simulink model "digitaltwin1c"  (R2020a)
settings: Solver=VariableStepAuto  StartTime=0.0  StopTime=stoptimetotal  RelTol=1e-3
values from neighbouring files (symbols this model uses):
  IC = load('params/IC_HoverAt10ftOcto.mat').IC    [prognostics.m]    (also in workspace_1.mat = )
  Motortwin1 = load('params/Motors/Motor1.mat').Motor    [prognostics.m]    (also in workspace_1.mat = )
  Motortwin2 = load('params/Motors/Motor2.mat').Motor    [prognostics.m]    (also in workspace_1.mat = )
  Motortwin3 = load('params/Motors/Motor3.mat').Motor    [prognostics.m]    (also in workspace_1.mat = )
  Motortwin4 = load('params/Motors/Motor4.mat').Motor    [prognostics.m]    (also in workspace_1.mat = )
  Motortwin5 = load('params/Motors/Motor5.mat').Motor    [prognostics.m]    (also in workspace_1.mat = )
  Motortwin6 = load('params/Motors/Motor6.mat').Motor    [prognostics.m]    (also in workspace_1.mat = )
  Motortwin7 = load('params/Motors/Motor7.mat').Motor    [prognostics.m]    (also in workspace_1.mat = )
  Motortwin8 = load('params/Motors/Motor8.mat').Motor    [prognostics.m]    (also in workspace_1.mat = )
  octomodel = load('params/octoModel.mat').octomodel    [prognostics.m]    (also in workspace_1.mat = )
  sampletimetraj = 1    [prognostics.m]    (also in workspace_1.mat)
undefined symbols (not defined in the file or in its folder): DiscIntNeverNeededParam, mu_wind
libraries: simulink x1, dspstat3 x1
(part 1 of 2)
settings Model: Creator=Researcher  LastModifiedBy=darrahts
settings DataIOCC: ReturnWorkspaceOutputs=off
settings DebuggingCC: ArithmeticOperatorsInVariantConditions=warning
settings SFSimCC: SimUseLocalCustomCode=off  CustomCodeUndefinedFunction=UseInterfaceOnly
settings RTWCC: RTWUseLocalCustomCode=off

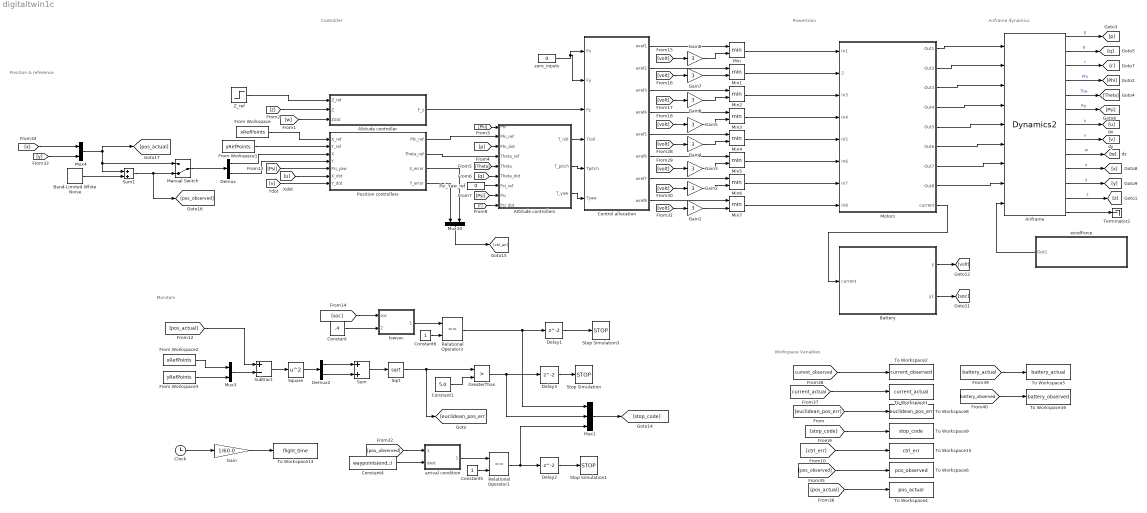
== system digitaltwin1c ==
  note: Workspace Variables
  note: Airframe dynamics
  note: Position & reference
  note: Controller
  note: Monitors
  note: Powertrain
  Airframe : M-S-Function  FunctionName=Dynamics2  Parameters=octomodel, IC
  Altitude controller : Subsystem
  Attitude controllers : Subsystem
  Band-Limited White Noise : simulink/Sources/Band-Limited White Noise  Cov=posNoise  Ts=sampletimetraj  seed=23
  Battery : Subsystem
  Clock : Clock
  Constant : Constant  Value=.4
  Constant1 : Constant  Value=5.0
  Constant4 : Constant  Value=waypoints(end,:)
  Constant5 : Constant
  Constant6 : Constant
  Control allocation : MATLAB Function  TreatAsAtomicUnit=on
  Delay1 : Delay
  Delay2 : Delay
  Delay3 : Delay
  Demux : Demux  Outputs=2
  Demux2 : Demux  Outputs=2
  From Workspace : FromWorkspace  VariableName=xRefPoints  SampleTime=sampletimetraj
  From Workspace1 : FromWorkspace  VariableName=yRefPoints  SampleTime=sampletimetraj
  From Workspace2 : FromWorkspace  VariableName=xRefPoints  SampleTime=sampletimetraj
  From Workspace3 : FromWorkspace  VariableName=yRefPoints  SampleTime=sampletimetraj
  Gain : Gain  Gain=1/60.0
  Gain{1..8} (8 alike) : Gain  Gain=3
  GreaterThan : RelationalOperator  Operator=>  OutDataTypeStr=boolean  RndMeth=Simplest
  Manual Switch : ManualSwitch  CurrentSetting=0
  Min{,1..7} (8 alike) : MinMax  Inputs=2
  Motors : Subsystem
  Mux1 : Mux  Inputs=3
  Mux10 : Mux  Inputs=2
  Mux3 : Mux  Inputs=2
  Mux4 : Mux  Inputs=2
  Position controllers : Subsystem
  Psi_Yaw_ref : Constant  Value=0
  Relational Operator1 : RelationalOperator  Operator===  OutDataTypeStr=boolean  RndMeth=Simplest
  Relational Operator3 : RelationalOperator  Operator===  OutDataTypeStr=boolean  RndMeth=Simplest
  Sqrt : Sqrt  SaturateOnIntegerOverflow=on
  Square : Math  Operator=square  SaturateOnIntegerOverflow=on
  Stop Simulation : Stop
  Stop Simulation1 : Stop
  Stop Simulation3 : Stop
  Subtract : Sum  Inputs=+-
  Sum : Sum
  Sum1 : Sum
  Terminator2 : Terminator
  To Workspace1 : ToWorkspace  VariableName=current_actual  SaveFormat=Timeseries  SampleTime=-1
  To Workspace13 : ToWorkspace  VariableName=flight_time  SaveFormat=Timeseries  SampleTime=-1
  To Workspace15 : ToWorkspace  VariableName=ctrl_err  SaveFormat=Timeseries  SampleTime=-1
  To Workspace16 : ToWorkspace  VariableName=battery_observed  SaveFormat=Timeseries  SampleTime=-1
  To Workspace2 : ToWorkspace  VariableName=current_observed  SaveFormat=Timeseries  SampleTime=-1
  To Workspace4 : ToWorkspace  VariableName=pos_actual  SaveFormat=Timeseries  SampleTime=-1
  To Workspace5 : ToWorkspace  VariableName=battery_actual  SaveFormat=Timeseries  SampleTime=-1
  To Workspace6 : ToWorkspace  VariableName=pos_observed  SaveFormat=Timeseries  SampleTime=-1
  To Workspace8 : ToWorkspace  VariableName=euclidean_pos_err  SaveFormat=Timeseries  SampleTime=-1
  To Workspace9 : ToWorkspace  VariableName=stop_code  SaveFormat=Timeseries  SampleTime=-1
  Z_ref : Step  Before=3  After=3  SampleTime=0
  arrival condition : MATLAB Function  TreatAsAtomicUnit=on
  lowsoc : MATLAB Function  TreatAsAtomicUnit=on
  windForce : Subsystem
  zero_inputs : Constant  Value=0
  wires:
  Airframe/1 -> [p]  "p"
  Airframe/2 -> [q]  "q"
  Airframe/3 -> [r]  "r"
  Airframe/4 -> [Phi]  "Phi"
  Airframe/5 -> [Theta]  "The"
  Airframe/6 -> [Psi]  "Psi"
  Airframe/11 -> [y]  "y"
  Airframe/12 -> [z]  "z"
  Airframe/7 -> [u]  "u"
  Airframe/10 -> [x]  "x"
  Airframe/9 -> [w]  "w"
  Airframe/8 -> [v]  "v"
  Motors/3(Out3) -> Airframe/3
  Motors/1(Out1) -> Airframe/1
  Motors/8(Out8) -> Airframe/8
  Motors/7(Out7) -> Airframe/7
  Motors/6(Out6) -> Airframe/6
  Motors/5(Out5) -> Airframe/5
  Motors/4(Out4) -> Airframe/4
  Motors/2(Out2) -> Airframe/2
  zero_inputs/1 -> Control allocation/1(Fx), Control allocation/2(Fy)
  Demux/2 -> Position controllers/4(Y)
  From Workspace1/1 -> Position controllers/2(Y_ref)
  From Workspace/1 -> Position controllers/1(X_ref)
  Demux/1 -> Position controllers/3(X)
  [Psi] -> Position controllers/5(Psi_yaw)
  [v] -> Position controllers/7(Y_dot)
  [u] -> Position controllers/6(X_dot)
  Position controllers/3(X_error) -> Mux10/2
  Position controllers/4(Y_error) -> Mux10/1
  Z_ref/1 -> Altitude controller/1(Z_ref)
  [z] -> Altitude controller/2(Z)
  Altitude controller/1(F_z) -> Control allocation/3(Fz)
  [Phi] -> Attitude controllers/1(Phi)
  [p] -> Attitude controllers/3(Phi_dot)
  Position controllers/2(Theta_ref) -> Attitude controllers/4(Theta_ref)
  [Theta] -> Attitude controllers/5(Theta)
  [q] -> Attitude controllers/6(Theta_dot)
  Psi_Yaw_ref/1 -> Attitude controllers/7(Psi_ref)
  [Psi] -> Attitude controllers/8(Psi)
  [r] -> Attitude controllers/9(Psi_dot)
  Attitude controllers/1(T_roll) -> Control allocation/4(Troll)
  Attitude controllers/2(T_pitch) -> Control allocation/5(Tpitch)
  Attitude controllers/3(T_yaw) -> Control allocation/6(Tyaw)
  Position controllers/1(Phi_ref) -> Attitude controllers/2(Phi_ref)
  [w] -> Altitude controller/3(Zdot)
  Airframe/13 -> Terminator2/1
  [volt] -> Gain1/1
  Min3/1 -> Motors/4(In4)
  Min4/1 -> Motors/5(In5)
  Min6/1 -> Motors/7(In7)
  Min7/1 -> Motors/8(In8)
  Control allocation/6(wref6) -> Min5/1
  Control allocation/7(wref7) -> Min6/1
  Gain4/1 -> Min4/2
  [volt] -> Gain8/1
  Min1/1 -> Motors/2(2)
  [volt] -> Gain3/1
  Control allocation/4(wref4) -> Min3/1
  [volt] -> Gain5/1
  [volt] -> Gain4/1
  Gain7/1 -> Min1/2
  Control allocation/2(wref2) -> Min1/1
  Gain5/1 -> Min3/2
  Min5/1 -> Motors/6(In6)
  Min2/1 -> Motors/3(In3)
  Min/1 -> Motors/1(In1)
  [volt] -> Gain6/1
  Control allocation/8(wref8) -> Min7/1
  Gain3/1 -> Min5/2
  [volt] -> Gain7/1
  Gain6/1 -> Min2/2
  Control allocation/1(wref1) -> Min/1
  Gain1/1 -> Min7/2
  Control allocation/3(wref3) -> Min2/1
  Gain2/1 -> Min6/2
  Gain8/1 -> Min/2
  [volt] -> Gain2/1
  Control allocation/5(wref5) -> Min4/1
  Mux4/1 -> [pos_actual], Manual Switch/1, Sum1/1
  [y] -> Mux4/2
  [x] -> Mux4/1
  Manual Switch/1 -> Demux/1
  Band-Limited White Noise/1 -> Sum1/2
  Sum1/1 -> [pos_observed], Manual Switch/2
  Clock/1 -> Gain/1
  Gain/1 -> To Workspace13/1
  Mux10/1 -> [ctrl_err]
  Motors/9(current) -> Battery/1(current)
  Battery/1(y) -> [volt]
  Battery/2(y1) -> [soc]
  windForce/1(Out1) -> Airframe/9
  Constant/1 -> lowsoc/2(threshold)
  From Workspace2/1 -> Mux3/1
  [soc] -> lowsoc/1(soc)
  Relational Operator1/1 -> Mux1/3, Delay2/1
  Sqrt/1 -> [euclidean_pos_err], GreaterThan/1
  Square/1 -> Demux2/1
  From Workspace3/1 -> Mux3/2
  Delay1/1 -> Stop Simulation3/1
  Mux1/1 -> [stop_code]
  Delay2/1 -> Stop Simulation1/1
  Constant1/1 -> GreaterThan/2
  GreaterThan/1 -> Mux1/2, Delay3/1
  Delay3/1 -> Stop Simulation/1
  [pos_observed] -> arrival condition/1(currentpos)
  Subtract/1 -> Square/1
  Demux2/2 -> Sum/2
  Constant6/1 -> Relational Operator3/2
  arrival condition/1(arrived) -> Relational Operator1/1
  Relational Operator3/1 -> Mux1/1, Delay1/1
  Sum/1 -> Sqrt/1
  Demux2/1 -> Sum/1
  Constant5/1 -> Relational Operator1/2
  Mux3/1 -> Subtract/2
  lowsoc/1(lowsoc) -> Relational Operator3/1
  [pos_actual] -> Subtract/1
  Constant4/1 -> arrival condition/2(dest)
  [euclidean_pos_err] -> To Workspace8/1
  [stop_code] -> To Workspace9/1
  [ctrl_err] -> To Workspace15/1
  [pos_observed] -> To Workspace6/1
  [pos_actual] -> To Workspace4/1
  [current_actual] -> To Workspace1/1
  [current_observed] -> To Workspace2/1
  [battery_actual] -> To Workspace5/1
  [battery_observed] -> To Workspace16/1

== system digitaltwin1c/Altitude controller ==
  Z_ref : Inport
  Z : Inport  Port=2
  Zdot : Inport  Port=3
  Add : Sum  Inputs=+++
  Add2 : Sum  Inputs=+-
  Constant2 : Constant  Value=octomodel.g*octomodel.mass
  Kdz : Gain  Gain=-3
  Kpz : Gain  Gain=-10
  mass : Gain  Gain=octomodel.mass
  mass1 : Gain  Gain=octomodel.mass
  F_z : Outport  VectorParamsAs1DForOutWhenUnconnected=off
  wires:
  Add2/1 -> Kpz/1
  Constant2/1 -> Add/1
  Z/1 -> Add2/1
  Add/1 -> F_z/1
  Z_ref/1 -> Add2/2
  Zdot/1 -> Kdz/1
  Kpz/1 -> mass/1
  Kdz/1 -> mass1/1
  mass1/1 -> Add/3
  mass/1 -> Add/2

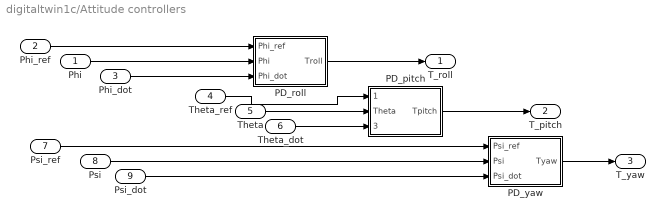
== system digitaltwin1c/Attitude controllers ==
  Phi : Inport
  Phi_ref : Inport  Port=2
  Phi_dot : Inport  Port=3
  Theta_ref : Inport  Port=4
  Theta : Inport  Port=5
  Theta_dot : Inport  Port=6
  Psi_ref : Inport  Port=7
  Psi : Inport  Port=8
  Psi_dot : Inport  Port=9
  PD_pitch : Subsystem
  PD_roll : Subsystem
  PD_yaw : Subsystem
  T_roll : Outport  VectorParamsAs1DForOutWhenUnconnected=off
  T_pitch : Outport  Port=2  VectorParamsAs1DForOutWhenUnconnected=off
  T_yaw : Outport  Port=3  VectorParamsAs1DForOutWhenUnconnected=off
  wires:
  PD_yaw/1(Tyaw) -> T_yaw/1
  PD_roll/1(Troll) -> T_roll/1
  Theta_ref/1 -> PD_pitch/1(Theta_ref)
  Theta_dot/1 -> PD_pitch/3(Theta_dot)
  PD_pitch/1(Tpitch) -> T_pitch/1
  Phi/1 -> PD_roll/2(Phi)
  Psi_dot/1 -> PD_yaw/3(Psi_dot)
  Psi_ref/1 -> PD_yaw/1(Psi_ref)
  Theta/1 -> PD_pitch/2(Theta)
  Phi_dot/1 -> PD_roll/3(Phi_dot)
  Psi/1 -> PD_yaw/2(Psi)
  Phi_ref/1 -> PD_roll/1(Phi_ref)

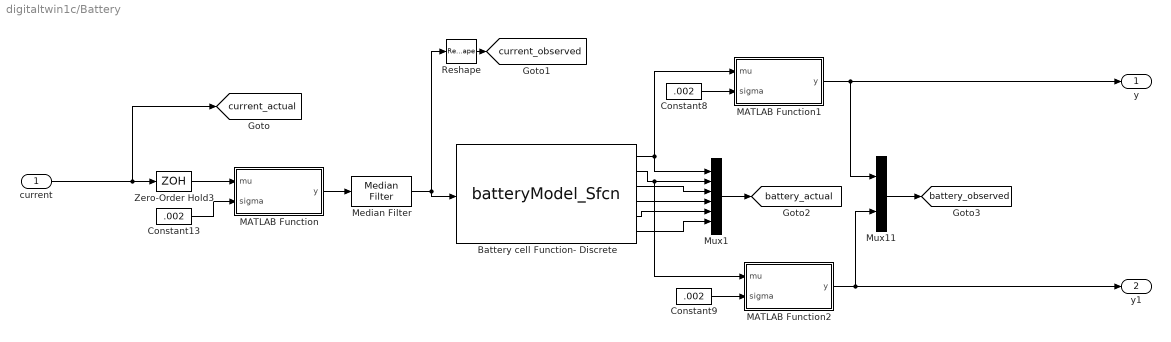
== system digitaltwin1c/Battery ==
  current : Inport
  Battery cell Function- Discrete : M-S-Function  FunctionName=batteryModel_Sfcn  Parameters=batterytwin, battery.dt
      mask Display:
      | port_label('input', 1, 'current');
      | port_label('output', 1, 'voltage');
      | port_label('output', 2, 'soc');
      | port_label('output', 3, 'R0');
      | port_label('output', 4, 'Ir');
      | port_label('output', 5, 'h');
      | port_label('output', 6, 'Q');
      | 
      | disp("Battery Cell");
  Constant13 : Constant  Value=.002
  Constant8 : Constant  Value=.002
  Constant9 : Constant  Value=.002
  MATLAB Function : MATLAB Function  TreatAsAtomicUnit=on
  MATLAB Function1 : MATLAB Function  TreatAsAtomicUnit=on
  MATLAB Function2 : MATLAB Function  TreatAsAtomicUnit=on
  Median Filter : dspstat3/Median Filter  WindowLength=5  SimulateUsing=Interpreted execution
      settings: SourceProductBaseCode=DS
  Mux1 : Mux  Inputs=6
  Mux11 : Mux  Inputs=2
  Reshape : Reshape
  Zero-Order Hold3 : ZeroOrderHold
  y : Outport
  y1 : Outport  Port=2
  tag scope: battery_actual=global, battery_observed=global, current_actual=global, current_observed=global
  wires:
  current/1 -> [current_actual], Zero-Order Hold3/1
  MATLAB Function/1(y) -> Median Filter/1
  Mux11/1 -> [battery_observed]
  MATLAB Function1/1(y) -> y/1, Mux11/1
  MATLAB Function2/1(y) -> y1/1, Mux11/2
  Battery cell Function- Discrete/1 -> MATLAB Function1/1(mu), Mux1/1
  Zero-Order Hold3/1 -> MATLAB Function/1(mu)
  Constant8/1 -> MATLAB Function1/2(sigma)
  Median Filter/1 -> Reshape/1, Battery cell Function- Discrete/1
  Battery cell Function- Discrete/2 -> MATLAB Function2/1(mu), Mux1/2
  Mux1/1 -> [battery_actual]
  Constant13/1 -> MATLAB Function/2(sigma)
  Constant9/1 -> MATLAB Function2/2(sigma)
  Battery cell Function- Discrete/3 -> Mux1/3
  Battery cell Function- Discrete/4 -> Mux1/4
  Battery cell Function- Discrete/5 -> Mux1/5
  Battery cell Function- Discrete/6 -> Mux1/6
  Reshape/1 -> [current_observed]

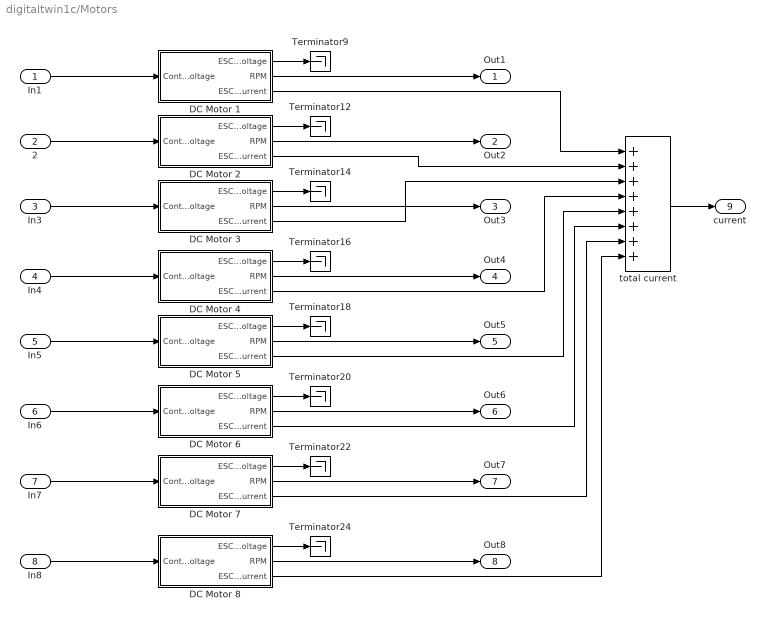
== system digitaltwin1c/Motors ==
  In1 : Inport
  2 : Inport  Port=2
  In3 : Inport  Port=3
  In4 : Inport  Port=4
  In5 : Inport  Port=5
  In6 : Inport  Port=6
  In7 : Inport  Port=7
  In8 : Inport  Port=8
  "DC Motor 1 " : Subsystem
  DC Motor 2 : Subsystem
  DC Motor 3 : Subsystem
  DC Motor 4 : Subsystem
  DC Motor 5 : Subsystem
  DC Motor 6 : Subsystem
  DC Motor 7 : Subsystem
  DC Motor 8 : Subsystem
  Terminator{9,12,14,16,18,20,22,24} (8 alike) : Terminator
  total current : Sum  Inputs=++++++++
  Out1 : Outport  VectorParamsAs1DForOutWhenUnconnected=off
  Out2 : Outport  Port=2  VectorParamsAs1DForOutWhenUnconnected=off
  Out3 : Outport  Port=3  VectorParamsAs1DForOutWhenUnconnected=off
  Out4 : Outport  Port=4  VectorParamsAs1DForOutWhenUnconnected=off
  Out5 : Outport  Port=5  VectorParamsAs1DForOutWhenUnconnected=off
  Out6 : Outport  Port=6  VectorParamsAs1DForOutWhenUnconnected=off
  Out7 : Outport  Port=7  VectorParamsAs1DForOutWhenUnconnected=off
  Out8 : Outport  Port=8  VectorParamsAs1DForOutWhenUnconnected=off
  current : Outport  Port=9  VectorParamsAs1DForOutWhenUnconnected=off
  wires:
  DC Motor 5/1(ESC Voltage) -> Terminator18/1
  DC Motor 6/3(ESC Current) -> total current/6
  DC Motor 7/3(ESC Current) -> total current/7
  DC Motor 7/1(ESC Voltage) -> Terminator22/1
  DC Motor 6/1(ESC Voltage) -> Terminator20/1
  DC Motor 5/3(ESC Current) -> total current/5
  DC Motor 8/3(ESC Current) -> total current/8
  "DC Motor 1 "/3(ESC Current) -> total current/1
  "DC Motor 1 "/1(ESC Voltage) -> Terminator9/1
  DC Motor 2/3(ESC Current) -> total current/2
  DC Motor 2/1(ESC Voltage) -> Terminator12/1
  DC Motor 3/1(ESC Voltage) -> Terminator14/1
  DC Motor 4/3(ESC Current) -> total current/4
  DC Motor 3/3(ESC Current) -> total current/3
  DC Motor 5/2(RPM) -> Out5/1
  DC Motor 4/1(ESC Voltage) -> Terminator16/1
  DC Motor 8/1(ESC Voltage) -> Terminator24/1
  DC Motor 7/2(RPM) -> Out7/1
  DC Motor 2/2(RPM) -> Out2/1
  DC Motor 3/2(RPM) -> Out3/1
  DC Motor 4/2(RPM) -> Out4/1
  DC Motor 6/2(RPM) -> Out6/1
  DC Motor 8/2(RPM) -> Out8/1
  "DC Motor 1 "/2(RPM) -> Out1/1
  In1/1 -> "DC Motor 1 "/1(Control  Voltage)
  In7/1 -> DC Motor 7/1(Control  Voltage)
  In8/1 -> DC Motor 8/1(Control  Voltage)
  In6/1 -> DC Motor 6/1(Control  Voltage)
  In5/1 -> DC Motor 5/1(Control  Voltage)
  In4/1 -> DC Motor 4/1(Control  Voltage)
  In3/1 -> DC Motor 3/1(Control  Voltage)
  2/1 -> DC Motor 2/1(Control  Voltage)
  total current/1 -> current/1

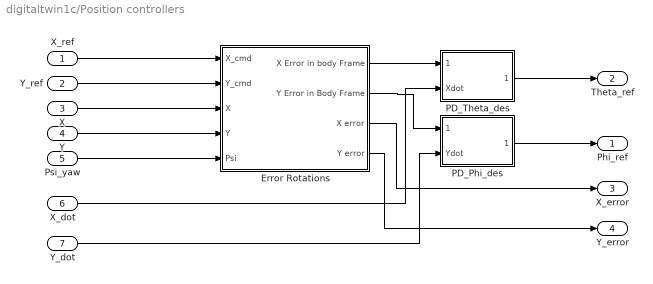
== system digitaltwin1c/Position controllers ==
  X_ref : Inport
  Y_ref : Inport  Port=2
  X : Inport  Port=3
  Y : Inport  Port=4
  Psi_yaw : Inport  Port=5
  X_dot : Inport  Port=6
  Y_dot : Inport  Port=7
  Error Rotations : Subsystem
  PD_Phi_des : Subsystem
  PD_Theta_des : Subsystem
  Phi_ref : Outport  VectorParamsAs1DForOutWhenUnconnected=off
  Theta_ref : Outport  Port=2  VectorParamsAs1DForOutWhenUnconnected=off
  X_error : Outport  Port=3  VectorParamsAs1DForOutWhenUnconnected=off
  Y_error : Outport  Port=4  VectorParamsAs1DForOutWhenUnconnected=off
  wires:
  Y/1 -> Error Rotations/4(Y)
  Y_ref/1 -> Error Rotations/2(Y_cmd)
  Error Rotations/4("Y error ") -> Y_error/1
  Error Rotations/3(X error) -> X_error/1
  Error Rotations/1(X Error in body Frame) -> PD_Theta_des/1(Xdot_ref)
  X/1 -> Error Rotations/3(X)
  Y_dot/1 -> PD_Phi_des/2(Ydot)
  PD_Phi_des/1(Phi_des) -> Phi_ref/1
  Error Rotations/2(Y Error in Body Frame) -> PD_Phi_des/1(Ydot_ref)
  Psi_yaw/1 -> Error Rotations/5(Psi)
  PD_Theta_des/1(Theta_des) -> Theta_ref/1
  X_dot/1 -> PD_Theta_des/2(Xdot)
  X_ref/1 -> Error Rotations/1(X_cmd)

== system digitaltwin1c/windForce ==
  Constant10 : Constant  Value=[0;0;0]
  Gain : Gain  Gain=.5
  Manual Switch1 : ManualSwitch  CurrentSetting=0
  Mux9 : Mux  Inputs=3
  Random Number : RandomNumber  Mean=mu_wind  Variance=.5  Seed=37
  Random Number1 : RandomNumber  Mean=mu_wind  Variance=.5  Seed=41
  Random Number2 : RandomNumber  Mean=mu_wind  Variance=.5
  Out1 : Outport
  wires:
  Random Number1/1 -> Mux9/2
  Mux9/1 -> Gain/1
  Manual Switch1/1 -> Out1/1
  Random Number2/1 -> Mux9/3
  Random Number/1 -> Mux9/1
  Constant10/1 -> Manual Switch1/1
  Gain/1 -> Manual Switch1/2

== system digitaltwin1c/Attitude controllers/PD_pitch ==
  Theta_ref : Inport
  Theta : Inport  Port=2
  Theta_dot : Inport  Port=3
  Add : Sum  Inputs=-+
  Gain : Gain  Gain=3
  Gain1 : Gain
  Gain2 : Gain  Gain=-1
  Sum : Sum  Inputs=|++
  Tpitch : Outport  VectorParamsAs1DForOutWhenUnconnected=off
  wires:
  Gain2/1 -> Tpitch/1
  Gain/1 -> Sum/1
  Theta/1 -> Add/2
  Add/1 -> Gain/1
  Gain1/1 -> Sum/2
  Sum/1 -> Gain2/1
  Theta_dot/1 -> Gain1/1
  Theta_ref/1 -> Add/1

== system digitaltwin1c/Attitude controllers/PD_roll ==
  Phi_ref : Inport
  Phi : Inport  Port=2
  Phi_dot : Inport  Port=3
  Add : Sum  Inputs=-+
  Gain : Gain  Gain=3
  Gain1 : Gain
  Gain2 : Gain  Gain=-1
  Sum : Sum  Inputs=|++
  Troll : Outport  VectorParamsAs1DForOutWhenUnconnected=off
  wires:
  Phi_ref/1 -> Add/1
  Phi_dot/1 -> Gain1/1
  Sum/1 -> Gain2/1
  Gain1/1 -> Sum/2
  Add/1 -> Gain/1
  Phi/1 -> Add/2
  Gain/1 -> Sum/1
  Gain2/1 -> Troll/1

== system digitaltwin1c/Attitude controllers/PD_yaw ==
  Psi_ref : Inport
  Psi : Inport  Port=2
  Psi_dot : Inport  Port=3
  Add : Sum  Inputs=-+
  Gain : Gain  Gain=3
  Gain1 : Gain
  Gain2 : Gain  Gain=-1
  Sum : Sum  Inputs=|++
  Tyaw : Outport  VectorParamsAs1DForOutWhenUnconnected=off
  wires:
  Psi_ref/1 -> Add/1
  Psi_dot/1 -> Gain1/1
  Sum/1 -> Gain2/1
  Gain1/1 -> Sum/2
  Add/1 -> Gain/1
  Psi/1 -> Add/2
  Gain/1 -> Sum/1
  Gain2/1 -> Tyaw/1

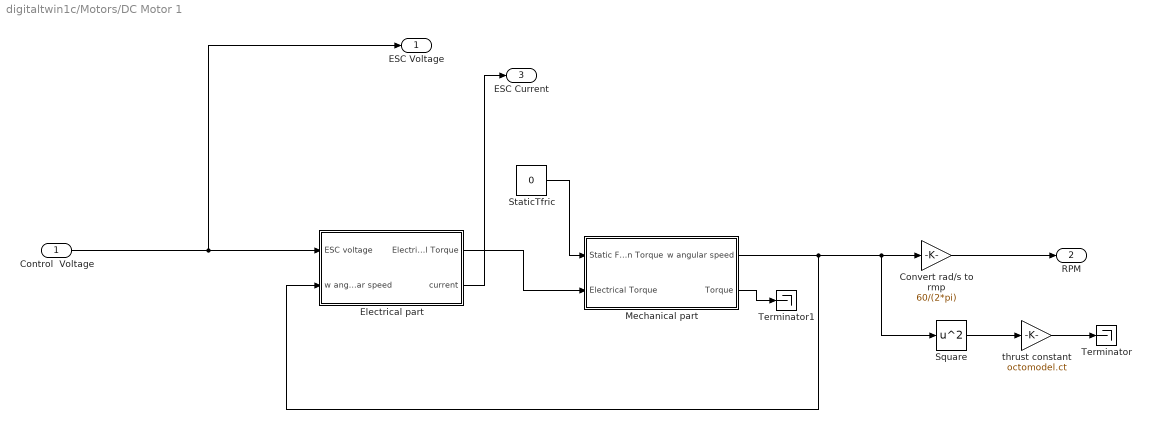
== system digitaltwin1c/Motors/DC Motor 1  ==
  Control  Voltage : Inport
  Convert rad/s to rmp : Gain  Gain=60/(2*pi)
  Electrical part : Subsystem
  Mechanical part : Subsystem
  Square : Math  Operator=square  SaturateOnIntegerOverflow=on
  StaticTfric : Constant  Value=0
  Terminator : Terminator
  Terminator1 : Terminator
  thrust constant : Gain  Gain=octomodel.ct
  ESC Voltage : Outport  VectorParamsAs1DForOutWhenUnconnected=off
  RPM : Outport  Port=2  VectorParamsAs1DForOutWhenUnconnected=off
  ESC Current : Outport  Port=3  VectorParamsAs1DForOutWhenUnconnected=off
  wires:
  Electrical part/1(Electrical Torque) -> Mechanical part/2(Electrical Torque)
  StaticTfric/1 -> Mechanical part/1(Static Friction Torque)
  Control  Voltage/1 -> ESC Voltage/1, Electrical part/1(ESC voltage)
  Electrical part/2(current) -> ESC Current/1
  Convert rad/s to rmp/1 -> RPM/1
  Mechanical part/1(w angular speed) -> Electrical part/2(w angular speed), Square/1, Convert rad/s to rmp/1
  Square/1 -> thrust constant/1
  thrust constant/1 -> Terminator/1
  Mechanical part/2(Torque) -> Terminator1/1

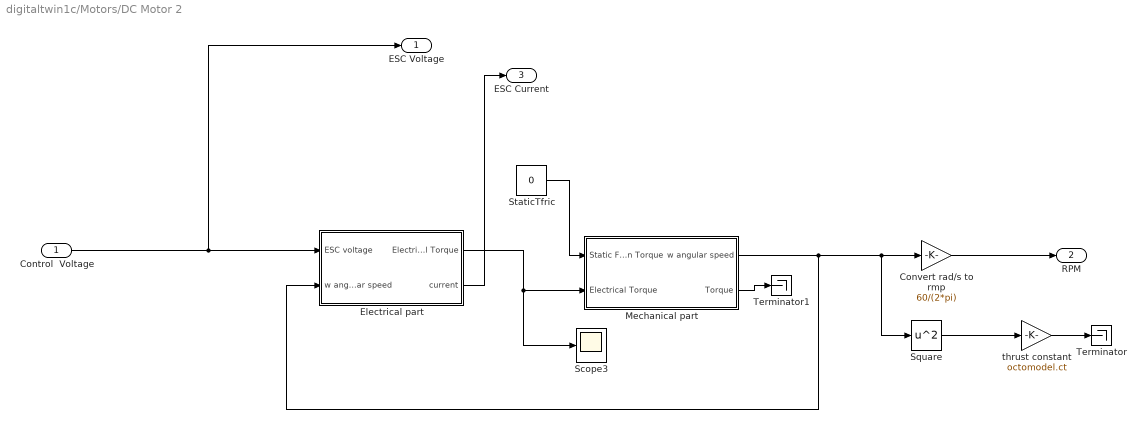
== system digitaltwin1c/Motors/DC Motor 2 ==
  Control  Voltage : Inport
  Convert rad/s to rmp : Gain  Gain=60/(2*pi)
  Electrical part : Subsystem
  Mechanical part : Subsystem
  Scope3 : Scope
  Square : Math  Operator=square  SaturateOnIntegerOverflow=on
  StaticTfric : Constant  Value=0
  Terminator : Terminator
  Terminator1 : Terminator
  thrust constant : Gain  Gain=octomodel.ct
  ESC Voltage : Outport  VectorParamsAs1DForOutWhenUnconnected=off
  RPM : Outport  Port=2  VectorParamsAs1DForOutWhenUnconnected=off
  ESC Current : Outport  Port=3  VectorParamsAs1DForOutWhenUnconnected=off
  wires:
  Square/1 -> thrust constant/1
  Mechanical part/1(w angular speed) -> Convert rad/s to rmp/1, Square/1, Electrical part/2(w angular speed)
  Convert rad/s to rmp/1 -> RPM/1
  Electrical part/2(current) -> ESC Current/1
  Control  Voltage/1 -> Electrical part/1(ESC voltage), ESC Voltage/1
  StaticTfric/1 -> Mechanical part/1(Static Friction Torque)
  Electrical part/1(Electrical Torque) -> Mechanical part/2(Electrical Torque), Scope3/1
  thrust constant/1 -> Terminator/1
  Mechanical part/2(Torque) -> Terminator1/1

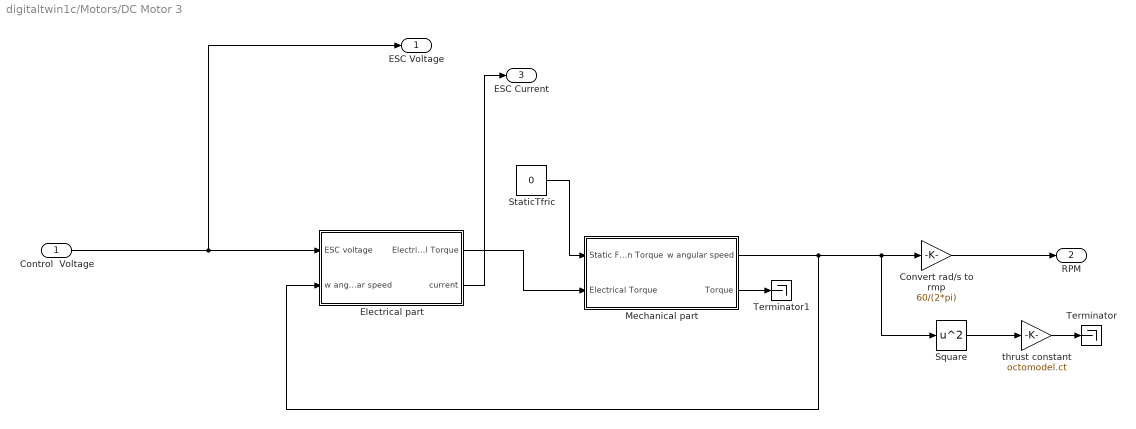
== system digitaltwin1c/Motors/DC Motor 3 ==
  Control  Voltage : Inport
  Convert rad/s to rmp : Gain  Gain=60/(2*pi)
  Electrical part : Subsystem
  Mechanical part : Subsystem
  Square : Math  Operator=square  SaturateOnIntegerOverflow=on
  StaticTfric : Constant  Value=0
  Terminator : Terminator
  Terminator1 : Terminator
  thrust constant : Gain  Gain=octomodel.ct
  ESC Voltage : Outport  VectorParamsAs1DForOutWhenUnconnected=off
  RPM : Outport  Port=2  VectorParamsAs1DForOutWhenUnconnected=off
  ESC Current : Outport  Port=3  VectorParamsAs1DForOutWhenUnconnected=off
  wires:
  Electrical part/1(Electrical Torque) -> Mechanical part/2(Electrical Torque)
  StaticTfric/1 -> Mechanical part/1(Static Friction Torque)
  Control  Voltage/1 -> ESC Voltage/1, Electrical part/1(ESC voltage)
  Electrical part/2(current) -> ESC Current/1
  Convert rad/s to rmp/1 -> RPM/1
  Mechanical part/1(w angular speed) -> Electrical part/2(w angular speed), Square/1, Convert rad/s to rmp/1
  Square/1 -> thrust constant/1
  thrust constant/1 -> Terminator/1
  Mechanical part/2(Torque) -> Terminator1/1

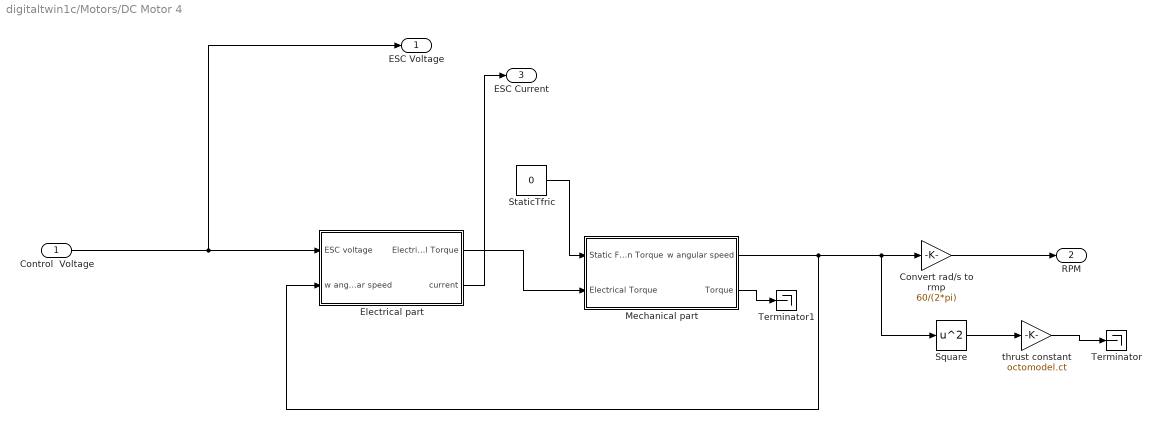
== system digitaltwin1c/Motors/DC Motor 4 ==
  Control  Voltage : Inport
  Convert rad/s to rmp : Gain  Gain=60/(2*pi)
  Electrical part : Subsystem
  Mechanical part : Subsystem
  Square : Math  Operator=square  SaturateOnIntegerOverflow=on
  StaticTfric : Constant  Value=0
  Terminator : Terminator
  Terminator1 : Terminator
  thrust constant : Gain  Gain=octomodel.ct
  ESC Voltage : Outport  VectorParamsAs1DForOutWhenUnconnected=off
  RPM : Outport  Port=2  VectorParamsAs1DForOutWhenUnconnected=off
  ESC Current : Outport  Port=3  VectorParamsAs1DForOutWhenUnconnected=off
  wires:
  Square/1 -> thrust constant/1
  Mechanical part/1(w angular speed) -> Convert rad/s to rmp/1, Square/1, Electrical part/2(w angular speed)
  Convert rad/s to rmp/1 -> RPM/1
  Electrical part/2(current) -> ESC Current/1
  Control  Voltage/1 -> Electrical part/1(ESC voltage), ESC Voltage/1
  StaticTfric/1 -> Mechanical part/1(Static Friction Torque)
  Electrical part/1(Electrical Torque) -> Mechanical part/2(Electrical Torque)
  thrust constant/1 -> Terminator/1
  Mechanical part/2(Torque) -> Terminator1/1

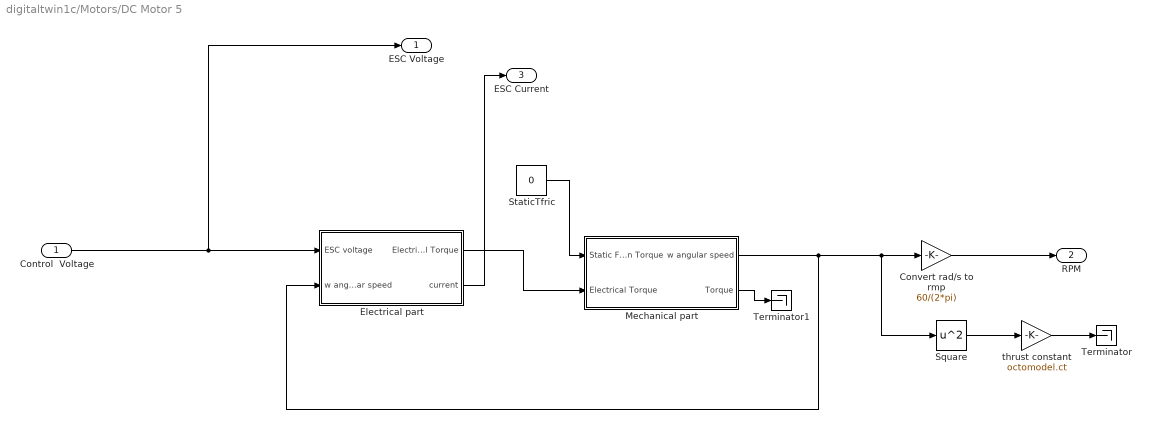
== system digitaltwin1c/Motors/DC Motor 5 ==
  Control  Voltage : Inport
  Convert rad/s to rmp : Gain  Gain=60/(2*pi)
  Electrical part : Subsystem
  Mechanical part : Subsystem
  Square : Math  Operator=square  SaturateOnIntegerOverflow=on
  StaticTfric : Constant  Value=0
  Terminator : Terminator
  Terminator1 : Terminator
  thrust constant : Gain  Gain=octomodel.ct
  ESC Voltage : Outport  VectorParamsAs1DForOutWhenUnconnected=off
  RPM : Outport  Port=2  VectorParamsAs1DForOutWhenUnconnected=off
  ESC Current : Outport  Port=3  VectorParamsAs1DForOutWhenUnconnected=off
  wires:
  Electrical part/1(Electrical Torque) -> Mechanical part/2(Electrical Torque)
  StaticTfric/1 -> Mechanical part/1(Static Friction Torque)
  Control  Voltage/1 -> ESC Voltage/1, Electrical part/1(ESC voltage)
  Electrical part/2(current) -> ESC Current/1
  Convert rad/s to rmp/1 -> RPM/1
  Mechanical part/1(w angular speed) -> Electrical part/2(w angular speed), Square/1, Convert rad/s to rmp/1
  Square/1 -> thrust constant/1
  thrust constant/1 -> Terminator/1
  Mechanical part/2(Torque) -> Terminator1/1

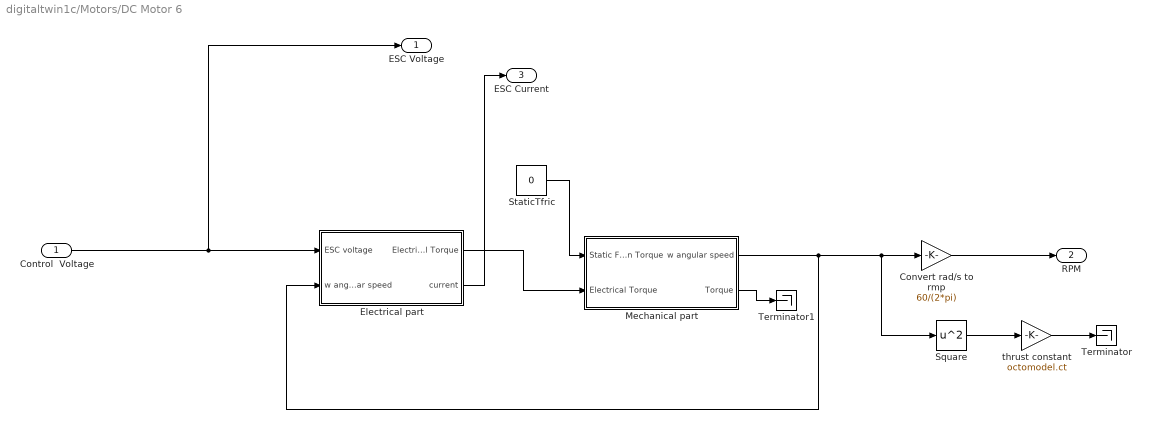
== system digitaltwin1c/Motors/DC Motor 6 ==
  Control  Voltage : Inport
  Convert rad/s to rmp : Gain  Gain=60/(2*pi)
  Electrical part : Subsystem
  Mechanical part : Subsystem
  Square : Math  Operator=square  SaturateOnIntegerOverflow=on
  StaticTfric : Constant  Value=0
  Terminator : Terminator
  Terminator1 : Terminator
  thrust constant : Gain  Gain=octomodel.ct
  ESC Voltage : Outport  VectorParamsAs1DForOutWhenUnconnected=off
  RPM : Outport  Port=2  VectorParamsAs1DForOutWhenUnconnected=off
  ESC Current : Outport  Port=3  VectorParamsAs1DForOutWhenUnconnected=off
  wires:
  Square/1 -> thrust constant/1
  Mechanical part/1(w angular speed) -> Convert rad/s to rmp/1, Square/1, Electrical part/2(w angular speed)
  Convert rad/s to rmp/1 -> RPM/1
  Electrical part/2(current) -> ESC Current/1
  Control  Voltage/1 -> Electrical part/1(ESC voltage), ESC Voltage/1
  StaticTfric/1 -> Mechanical part/1(Static Friction Torque)
  Electrical part/1(Electrical Torque) -> Mechanical part/2(Electrical Torque)
  thrust constant/1 -> Terminator/1
  Mechanical part/2(Torque) -> Terminator1/1

== system digitaltwin1c/Motors/DC Motor 7 ==
  Control  Voltage : Inport
  Convert rad/s to rmp : Gain  Gain=60/(2*pi)
  Electrical part : Subsystem
  Mechanical part : Subsystem
  Square : Math  Operator=square  SaturateOnIntegerOverflow=on
  StaticTfric : Constant  Value=0
  Terminator : Terminator
  Terminator1 : Terminator
  thrust constant : Gain  Gain=octomodel.ct
  ESC Voltage : Outport  VectorParamsAs1DForOutWhenUnconnected=off
  RPM : Outport  Port=2  VectorParamsAs1DForOutWhenUnconnected=off
  ESC Current : Outport  Port=3  VectorParamsAs1DForOutWhenUnconnected=off
  wires:
  Electrical part/1(Electrical Torque) -> Mechanical part/2(Electrical Torque)
  StaticTfric/1 -> Mechanical part/1(Static Friction Torque)
  Control  Voltage/1 -> ESC Voltage/1, Electrical part/1(ESC voltage)
  Electrical part/2(current) -> ESC Current/1
  Convert rad/s to rmp/1 -> RPM/1
  Mechanical part/1(w angular speed) -> Electrical part/2(w angular speed), Square/1, Convert rad/s to rmp/1
  Square/1 -> thrust constant/1
  thrust constant/1 -> Terminator/1
  Mechanical part/2(Torque) -> Terminator1/1

== system digitaltwin1c/Motors/DC Motor 8 ==
  Control  Voltage : Inport
  Convert rad/s to rmp : Gain  Gain=60/(2*pi)
  Electrical part : Subsystem
  Mechanical part : Subsystem
  Square : Math  Operator=square  SaturateOnIntegerOverflow=on
  StaticTfric : Constant  Value=0
  Terminator : Terminator
  Terminator1 : Terminator
  thrust constant : Gain  Gain=octomodel.ct
  ESC Voltage : Outport  VectorParamsAs1DForOutWhenUnconnected=off
  RPM : Outport  Port=2  VectorParamsAs1DForOutWhenUnconnected=off
  ESC Current : Outport  Port=3  VectorParamsAs1DForOutWhenUnconnected=off
  wires:
  Square/1 -> thrust constant/1
  Mechanical part/1(w angular speed) -> Convert rad/s to rmp/1, Square/1, Electrical part/2(w angular speed)
  Convert rad/s to rmp/1 -> RPM/1
  Electrical part/2(current) -> ESC Current/1
  Control  Voltage/1 -> Electrical part/1(ESC voltage), ESC Voltage/1
  StaticTfric/1 -> Mechanical part/1(Static Friction Torque)
  Electrical part/1(Electrical Torque) -> Mechanical part/2(Electrical Torque)
  thrust constant/1 -> Terminator/1
  Mechanical part/2(Torque) -> Terminator1/1

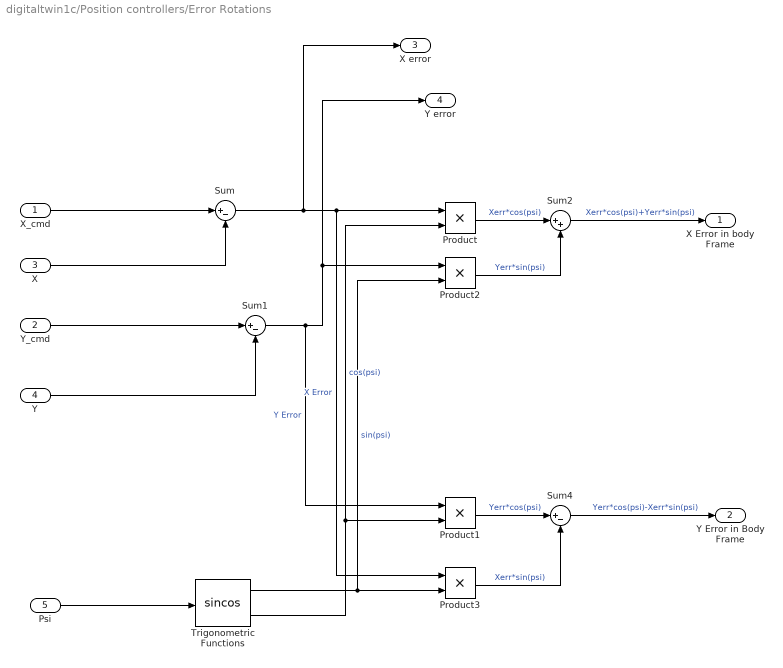
== system digitaltwin1c/Position controllers/Error Rotations ==
  X_cmd : Inport
  Y_cmd : Inport  Port=2
  X : Inport  Port=3
  Y : Inport  Port=4
  Psi : Inport  Port=5
  Product{,1..3} (4 alike) : Product
  Sum : Sum  Inputs=|+-
  Sum1 : Sum  Inputs=|+-
  Sum2 : Sum  Inputs=|++
  Sum4 : Sum  Inputs=|+-
  Trigonometric Functions : Trigonometry  Operator=sincos
  X Error in body Frame : Outport  VectorParamsAs1DForOutWhenUnconnected=off
  Y Error in Body Frame : Outport  Port=2  VectorParamsAs1DForOutWhenUnconnected=off
  X error : Outport  Port=3  VectorParamsAs1DForOutWhenUnconnected=off
  "Y error " : Outport  Port=4  VectorParamsAs1DForOutWhenUnconnected=off
  wires:
  Sum4/1 -> Y Error in Body Frame/1  "Yerr*cos(psi)-Xerr*sin(psi)"
  Product3/1 -> Sum4/2  "Xerr*sin(psi)"
  Sum1/1 -> "Y error "/1, Product2/1, Product1/1  "Y Error"
  Trigonometric Functions/1 -> Product2/2, Product3/2  "sin(psi)"
  Sum2/1 -> X Error in body Frame/1  "Xerr*cos(psi)+Yerr*sin(psi)"
  Y_cmd/1 -> Sum1/1
  X_cmd/1 -> Sum/1
  X/1 -> Sum/2
  Y/1 -> Sum1/2
  Sum/1 -> X error/1, Product3/1, Product/1  "X Error"
  Trigonometric Functions/2 -> Product/2, Product1/2  "cos(psi)"
  Product/1 -> Sum2/1  "Xerr*cos(psi)"
  Product2/1 -> Sum2/2  "Yerr*sin(psi)"
  Product1/1 -> Sum4/1  "Yerr*cos(psi)"
  Psi/1 -> Trigonometric Functions/1

== system digitaltwin1c/Position controllers/PD_Phi_des ==
  Ydot_ref : Inport
  Ydot : Inport  Port=2
  Add : Sum  Inputs=+-
  Gain : Gain  Gain=0.1
  Gain1 : Gain  Gain=0
  Gain2 : Gain  Gain=-1
  Saturation in radians : Saturate  UpperLimit=12*pi/180  LowerLimit=-12*pi/180
  Sum : Sum  Inputs=|+-
  Phi_des : Outport  VectorParamsAs1DForOutWhenUnconnected=off
  wires:
  Saturation in radians/1 -> Phi_des/1
  Ydot_ref/1 -> Add/1
  Ydot/1 -> Add/2, Gain1/1
  Gain1/1 -> Sum/2
  Add/1 -> Gain/1
  Gain/1 -> Sum/1
  Sum/1 -> Gain2/1
  Gain2/1 -> Saturation in radians/1

== system digitaltwin1c/Position controllers/PD_Theta_des ==
  Xdot_ref : Inport
  Xdot : Inport  Port=2
  Add : Sum  Inputs=+-
  Gain : Gain  Gain=0.1
  Gain1 : Gain  Gain=0
  Saturation in radians : Saturate  UpperLimit=12*pi/180  LowerLimit=-12*pi/180
  Sum : Sum  Inputs=|+-
  Theta_des : Outport  VectorParamsAs1DForOutWhenUnconnected=off
  wires:
  Sum/1 -> Saturation in radians/1
  Gain/1 -> Sum/1
  Add/1 -> Gain/1
  Gain1/1 -> Sum/2
  Xdot/1 -> Gain1/1, Add/2
  Xdot_ref/1 -> Add/1
  Saturation in radians/1 -> Theta_des/1

== system digitaltwin1c/Motors/DC Motor 1 /Electrical part ==
  ESC voltage : Inport
  w angular speed : Inport  Port=2
  1/R : Gain  Gain=1/Motortwin1.Req
  Ke (Torque constant)1 : Gain  Gain=Motortwin1.Ke_eq
  Kt (Torque constant) Kt=Ke for an ideal square wave motor : Gain  Gain=Motortwin1.Ke_eq
  Saturation : Saturate  UpperLimit=11  LowerLimit=0
  Sum : Sum  Inputs=|+-
  Electrical Torque : Outport  VectorParamsAs1DForOutWhenUnconnected=off
  current : Outport  Port=2  VectorParamsAs1DForOutWhenUnconnected=off
  wires:
  1/R/1 -> Saturation/1  "current i"
  Sum/1 -> 1/R/1
  Kt (Torque constant) Kt=Ke for an ideal square wave motor/1 -> Electrical Torque/1
  Ke (Torque constant)1/1 -> Sum/2
  ESC voltage/1 -> Sum/1
  w angular speed/1 -> Ke (Torque constant)1/1
  Saturation/1 -> Kt (Torque constant) Kt=Ke for an ideal square wave motor/1, current/1

== system digitaltwin1c/Motors/DC Motor 1 /Mechanical part ==
  Static Friction Torque : Inport
  Electrical Torque : Inport  Port=2
  1/J Inertia constant : Gain  Gain=1/Motortwin1.J
  "Df viscous damping coefficient Dynamic Friction coefficient " : Gain  Gain=Motortwin1.Df
  Discrete-Time Integrator : DiscreteIntegrator  gainval=1  InitialCondition=IC.w1  SampleTime=octomodel.sampletime  ICPrevOutput=DiscIntNeverNeededParam  ICPrevScaledInput=DiscIntNeverNeededParam
  Gain : Gain  Gain=Motortwin1.cq
  Square : Math  Operator=square  SaturateOnIntegerOverflow=on
  Sum1 : Sum  Inputs=--+-
  w angular speed : Outport  VectorParamsAs1DForOutWhenUnconnected=off
  Torque : Outport  Port=2  VectorParamsAs1DForOutWhenUnconnected=off
  wires:
  1/J Inertia constant/1 -> Discrete-Time Integrator/1
  Static Friction Torque/1 -> Sum1/2
  "Df viscous damping coefficient Dynamic Friction coefficient "/1 -> Sum1/4
  Discrete-Time Integrator/1 -> w angular speed/1, Square/1, "Df viscous damping coefficient Dynamic Friction coefficient "/1  "w angular speed"
  Sum1/1 -> 1/J Inertia constant/1
  Electrical Torque/1 -> Sum1/3
  Gain/1 -> Torque/1, Sum1/1
  Square/1 -> Gain/1

== system digitaltwin1c/Motors/DC Motor 2/Electrical part ==
  ESC voltage : Inport
  w angular speed : Inport  Port=2
  1/R : Gain  Gain=1/Motortwin2.Req
  Ke (Torque constant)1 : Gain  Gain=Motortwin2.Ke_eq
  Kt (Torque constant) Kt=Ke for an ideal square wave motor : Gain  Gain=Motortwin2.Ke_eq
  Saturation : Saturate  UpperLimit=11  LowerLimit=0
  Sum : Sum  Inputs=|+-
  Electrical Torque : Outport  VectorParamsAs1DForOutWhenUnconnected=off
  current : Outport  Port=2  VectorParamsAs1DForOutWhenUnconnected=off
  wires:
  Saturation/1 -> current/1, Kt (Torque constant) Kt=Ke for an ideal square wave motor/1
  w angular speed/1 -> Ke (Torque constant)1/1
  ESC voltage/1 -> Sum/1
  Ke (Torque constant)1/1 -> Sum/2
  Kt (Torque constant) Kt=Ke for an ideal square wave motor/1 -> Electrical Torque/1
  Sum/1 -> 1/R/1
  1/R/1 -> Saturation/1  "current i"

== system digitaltwin1c/Motors/DC Motor 2/Mechanical part ==
  Static Friction Torque : Inport
  Electrical Torque : Inport  Port=2
  1/J Inertia constant : Gain  Gain=1/Motortwin2.J
  "Df viscous damping coefficient Dynamic Friction coefficient " : Gain  Gain=Motortwin2.Df
  Discrete-Time Integrator : DiscreteIntegrator  gainval=1  InitialCondition=IC.w2  SampleTime=octomodel.sampletime  ICPrevOutput=DiscIntNeverNeededParam  ICPrevScaledInput=DiscIntNeverNeededParam
  Gain : Gain  Gain=Motortwin2.cq
  Square : Math  Operator=square  SaturateOnIntegerOverflow=on
  Sum1 : Sum  Inputs=--+-
  w angular speed : Outport  VectorParamsAs1DForOutWhenUnconnected=off
  Torque : Outport  Port=2  VectorParamsAs1DForOutWhenUnconnected=off
  wires:
  Square/1 -> Gain/1
  Gain/1 -> Sum1/1, Torque/1
  Electrical Torque/1 -> Sum1/3
  Sum1/1 -> 1/J Inertia constant/1
  Discrete-Time Integrator/1 -> "Df viscous damping coefficient Dynamic Friction coefficient "/1, Square/1, w angular speed/1  "w angular speed"
  "Df viscous damping coefficient Dynamic Friction coefficient "/1 -> Sum1/4
  Static Friction Torque/1 -> Sum1/2
  1/J Inertia constant/1 -> Discrete-Time Integrator/1

== system digitaltwin1c/Motors/DC Motor 3/Electrical part ==
  ESC voltage : Inport
  w angular speed : Inport  Port=2
  1/R : Gain  Gain=1/Motortwin3.Req
  Ke (Torque constant)1 : Gain  Gain=Motortwin3.Ke_eq
  Kt (Torque constant) Kt=Ke for an ideal square wave motor : Gain  Gain=Motortwin3.Ke_eq
  Saturation : Saturate  UpperLimit=11  LowerLimit=0
  Sum : Sum  Inputs=|+-
  Electrical Torque : Outport  VectorParamsAs1DForOutWhenUnconnected=off
  current : Outport  Port=2  VectorParamsAs1DForOutWhenUnconnected=off
  wires:
  1/R/1 -> Saturation/1  "current i"
  Sum/1 -> 1/R/1
  Kt (Torque constant) Kt=Ke for an ideal square wave motor/1 -> Electrical Torque/1
  Ke (Torque constant)1/1 -> Sum/2
  ESC voltage/1 -> Sum/1
  w angular speed/1 -> Ke (Torque constant)1/1
  Saturation/1 -> Kt (Torque constant) Kt=Ke for an ideal square wave motor/1, current/1

== system digitaltwin1c/Motors/DC Motor 3/Mechanical part ==
  Static Friction Torque : Inport
  Electrical Torque : Inport  Port=2
  1/J Inertia constant : Gain  Gain=1/Motortwin3.J
  "Df viscous damping coefficient Dynamic Friction coefficient " : Gain  Gain=Motortwin3.Df
  Discrete-Time Integrator : DiscreteIntegrator  gainval=1  InitialCondition=IC.w3  SampleTime=octomodel.sampletime  ICPrevOutput=DiscIntNeverNeededParam  ICPrevScaledInput=DiscIntNeverNeededParam
  Gain : Gain  Gain=Motortwin3.cq
  Square : Math  Operator=square  SaturateOnIntegerOverflow=on
  Sum1 : Sum  Inputs=--+-
  w angular speed : Outport  VectorParamsAs1DForOutWhenUnconnected=off
  Torque : Outport  Port=2  VectorParamsAs1DForOutWhenUnconnected=off
  wires:
  1/J Inertia constant/1 -> Discrete-Time Integrator/1
  Static Friction Torque/1 -> Sum1/2
  "Df viscous damping coefficient Dynamic Friction coefficient "/1 -> Sum1/4
  Discrete-Time Integrator/1 -> w angular speed/1, Square/1, "Df viscous damping coefficient Dynamic Friction coefficient "/1  "w angular speed"
  Sum1/1 -> 1/J Inertia constant/1
  Electrical Torque/1 -> Sum1/3
  Gain/1 -> Torque/1, Sum1/1
  Square/1 -> Gain/1

== system digitaltwin1c/Motors/DC Motor 4/Electrical part ==
  ESC voltage : Inport
  w angular speed : Inport  Port=2
  1/R : Gain  Gain=1/Motortwin4.Req
  Ke (Torque constant)1 : Gain  Gain=Motortwin4.Ke_eq
  Kt (Torque constant) Kt=Ke for an ideal square wave motor : Gain  Gain=Motortwin4.Ke_eq
  Saturation : Saturate  UpperLimit=11  LowerLimit=0
  Sum : Sum  Inputs=|+-
  Electrical Torque : Outport  VectorParamsAs1DForOutWhenUnconnected=off
  current : Outport  Port=2  VectorParamsAs1DForOutWhenUnconnected=off
  wires:
  Saturation/1 -> current/1, Kt (Torque constant) Kt=Ke for an ideal square wave motor/1
  w angular speed/1 -> Ke (Torque constant)1/1
  ESC voltage/1 -> Sum/1
  Ke (Torque constant)1/1 -> Sum/2
  Kt (Torque constant) Kt=Ke for an ideal square wave motor/1 -> Electrical Torque/1
  Sum/1 -> 1/R/1
  1/R/1 -> Saturation/1  "current i"

== system digitaltwin1c/Motors/DC Motor 4/Mechanical part ==
  Static Friction Torque : Inport
  Electrical Torque : Inport  Port=2
  1/J Inertia constant : Gain  Gain=1/Motortwin4.J
  "Df viscous damping coefficient Dynamic Friction coefficient " : Gain  Gain=Motortwin4.Df
  Discrete-Time Integrator : DiscreteIntegrator  gainval=1  InitialCondition=IC.w4  SampleTime=octomodel.sampletime  ICPrevOutput=DiscIntNeverNeededParam  ICPrevScaledInput=DiscIntNeverNeededParam
  Gain : Gain  Gain=Motortwin4.cq
  Square : Math  Operator=square  SaturateOnIntegerOverflow=on
  Sum1 : Sum  Inputs=--+-
  w angular speed : Outport  VectorParamsAs1DForOutWhenUnconnected=off
  Torque : Outport  Port=2  VectorParamsAs1DForOutWhenUnconnected=off
  wires:
  Square/1 -> Gain/1
  Gain/1 -> Sum1/1, Torque/1
  Electrical Torque/1 -> Sum1/3
  Sum1/1 -> 1/J Inertia constant/1
  Discrete-Time Integrator/1 -> "Df viscous damping coefficient Dynamic Friction coefficient "/1, Square/1, w angular speed/1  "w angular speed"
  "Df viscous damping coefficient Dynamic Friction coefficient "/1 -> Sum1/4
  Static Friction Torque/1 -> Sum1/2
  1/J Inertia constant/1 -> Discrete-Time Integrator/1

== system digitaltwin1c/Motors/DC Motor 5/Electrical part ==
  ESC voltage : Inport
  w angular speed : Inport  Port=2
  1/R : Gain  Gain=1/Motortwin5.Req
  Ke (Torque constant)1 : Gain  Gain=Motortwin5.Ke_eq
  Kt (Torque constant) Kt=Ke for an ideal square wave motor : Gain  Gain=Motortwin5.Ke_eq
  Saturation : Saturate  UpperLimit=11  LowerLimit=0
  Sum : Sum  Inputs=|+-
  Electrical Torque : Outport  VectorParamsAs1DForOutWhenUnconnected=off
  current : Outport  Port=2  VectorParamsAs1DForOutWhenUnconnected=off
  wires:
  1/R/1 -> Saturation/1  "current i"
  Sum/1 -> 1/R/1
  Kt (Torque constant) Kt=Ke for an ideal square wave motor/1 -> Electrical Torque/1
  Ke (Torque constant)1/1 -> Sum/2
  ESC voltage/1 -> Sum/1
  w angular speed/1 -> Ke (Torque constant)1/1
  Saturation/1 -> Kt (Torque constant) Kt=Ke for an ideal square wave motor/1, current/1

== system digitaltwin1c/Motors/DC Motor 5/Mechanical part ==
  Static Friction Torque : Inport
  Electrical Torque : Inport  Port=2
  1/J Inertia constant : Gain  Gain=1/Motortwin5.J
  "Df viscous damping coefficient Dynamic Friction coefficient " : Gain  Gain=Motortwin5.Df
  Discrete-Time Integrator : DiscreteIntegrator  gainval=1  InitialCondition=IC.w5  SampleTime=octomodel.sampletime  ICPrevOutput=DiscIntNeverNeededParam  ICPrevScaledInput=DiscIntNeverNeededParam
  Gain : Gain  Gain=Motortwin5.cq
  Square : Math  Operator=square  SaturateOnIntegerOverflow=on
  Sum1 : Sum  Inputs=--+-
  w angular speed : Outport  VectorParamsAs1DForOutWhenUnconnected=off
  Torque : Outport  Port=2  VectorParamsAs1DForOutWhenUnconnected=off
  wires:
  1/J Inertia constant/1 -> Discrete-Time Integrator/1
  Static Friction Torque/1 -> Sum1/2
  "Df viscous damping coefficient Dynamic Friction coefficient "/1 -> Sum1/4
  Discrete-Time Integrator/1 -> w angular speed/1, Square/1, "Df viscous damping coefficient Dynamic Friction coefficient "/1  "w angular speed"
  Sum1/1 -> 1/J Inertia constant/1
  Electrical Torque/1 -> Sum1/3
  Gain/1 -> Torque/1, Sum1/1
  Square/1 -> Gain/1

== system digitaltwin1c/Motors/DC Motor 6/Electrical part ==
  ESC voltage : Inport
  w angular speed : Inport  Port=2
  1/R : Gain  Gain=1/Motortwin6.Req
  Ke (Torque constant)1 : Gain  Gain=Motortwin6.Ke_eq
  Kt (Torque constant) Kt=Ke for an ideal square wave motor : Gain  Gain=Motortwin6.Ke_eq
  Saturation : Saturate  UpperLimit=11  LowerLimit=0
  Sum : Sum  Inputs=|+-
  Electrical Torque : Outport  VectorParamsAs1DForOutWhenUnconnected=off
  current : Outport  Port=2  VectorParamsAs1DForOutWhenUnconnected=off
  wires:
  Saturation/1 -> current/1, Kt (Torque constant) Kt=Ke for an ideal square wave motor/1
  w angular speed/1 -> Ke (Torque constant)1/1
  ESC voltage/1 -> Sum/1
  Ke (Torque constant)1/1 -> Sum/2
  Kt (Torque constant) Kt=Ke for an ideal square wave motor/1 -> Electrical Torque/1
  Sum/1 -> 1/R/1
  1/R/1 -> Saturation/1  "current i"

== system digitaltwin1c/Motors/DC Motor 6/Mechanical part ==
  Static Friction Torque : Inport
  Electrical Torque : Inport  Port=2
  1/J Inertia constant : Gain  Gain=1/Motortwin6.J
  "Df viscous damping coefficient Dynamic Friction coefficient " : Gain  Gain=Motortwin6.Df
  Discrete-Time Integrator : DiscreteIntegrator  gainval=1  InitialCondition=IC.w6  SampleTime=octomodel.sampletime  ICPrevOutput=DiscIntNeverNeededParam  ICPrevScaledInput=DiscIntNeverNeededParam
  Gain : Gain  Gain=Motortwin6.cq
  Square : Math  Operator=square  SaturateOnIntegerOverflow=on
  Sum1 : Sum  Inputs=--+-
  w angular speed : Outport  VectorParamsAs1DForOutWhenUnconnected=off
  Torque : Outport  Port=2  VectorParamsAs1DForOutWhenUnconnected=off
  wires:
  Square/1 -> Gain/1
  Gain/1 -> Sum1/1, Torque/1
  Electrical Torque/1 -> Sum1/3
  Sum1/1 -> 1/J Inertia constant/1
  Discrete-Time Integrator/1 -> "Df viscous damping coefficient Dynamic Friction coefficient "/1, Square/1, w angular speed/1  "w angular speed"
  "Df viscous damping coefficient Dynamic Friction coefficient "/1 -> Sum1/4
  Static Friction Torque/1 -> Sum1/2
  1/J Inertia constant/1 -> Discrete-Time Integrator/1

== system digitaltwin1c/Motors/DC Motor 7/Electrical part ==
  ESC voltage : Inport
  w angular speed : Inport  Port=2
  1/R : Gain  Gain=1/Motortwin7.Req
  Ke (Torque constant)1 : Gain  Gain=Motortwin7.Ke_eq
  Kt (Torque constant) Kt=Ke for an ideal square wave motor : Gain  Gain=Motortwin7.Ke_eq
  Saturation : Saturate  UpperLimit=11  LowerLimit=0
  Sum : Sum  Inputs=|+-
  Electrical Torque : Outport  VectorParamsAs1DForOutWhenUnconnected=off
  current : Outport  Port=2  VectorParamsAs1DForOutWhenUnconnected=off
  wires:
  1/R/1 -> Saturation/1  "current i"
  Sum/1 -> 1/R/1
  Kt (Torque constant) Kt=Ke for an ideal square wave motor/1 -> Electrical Torque/1
  Ke (Torque constant)1/1 -> Sum/2
  ESC voltage/1 -> Sum/1
  w angular speed/1 -> Ke (Torque constant)1/1
  Saturation/1 -> Kt (Torque constant) Kt=Ke for an ideal square wave motor/1, current/1

== system digitaltwin1c/Motors/DC Motor 7/Mechanical part ==
  Static Friction Torque : Inport
  Electrical Torque : Inport  Port=2
  1/J Inertia constant : Gain  Gain=1/Motortwin7.J
  "Df viscous damping coefficient Dynamic Friction coefficient " : Gain  Gain=Motortwin7.Df
  Discrete-Time Integrator : DiscreteIntegrator  gainval=1  InitialCondition=IC.w7  SampleTime=octomodel.sampletime  ICPrevOutput=DiscIntNeverNeededParam  ICPrevScaledInput=DiscIntNeverNeededParam
  Gain : Gain  Gain=Motortwin7.cq
  Square : Math  Operator=square  SaturateOnIntegerOverflow=on
  Sum1 : Sum  Inputs=--+-
  w angular speed : Outport  VectorParamsAs1DForOutWhenUnconnected=off
  Torque : Outport  Port=2  VectorParamsAs1DForOutWhenUnconnected=off
  wires:
  1/J Inertia constant/1 -> Discrete-Time Integrator/1
  Static Friction Torque/1 -> Sum1/2
  "Df viscous damping coefficient Dynamic Friction coefficient "/1 -> Sum1/4
  Discrete-Time Integrator/1 -> w angular speed/1, Square/1, "Df viscous damping coefficient Dynamic Friction coefficient "/1  "w angular speed"
  Sum1/1 -> 1/J Inertia constant/1
  Electrical Torque/1 -> Sum1/3
  Gain/1 -> Torque/1, Sum1/1
  Square/1 -> Gain/1

== system digitaltwin1c/Motors/DC Motor 8/Electrical part ==
  ESC voltage : Inport
  w angular speed : Inport  Port=2
  1/R : Gain  Gain=1/Motortwin8.Req
  Ke (Torque constant)1 : Gain  Gain=Motortwin8.Ke_eq
  Kt (Torque constant) Kt=Ke for an ideal square wave motor : Gain  Gain=Motortwin8.Ke_eq
  Saturation : Saturate  UpperLimit=11  LowerLimit=0
  Sum : Sum  Inputs=|+-
  Electrical Torque : Outport  VectorParamsAs1DForOutWhenUnconnected=off
  current : Outport  Port=2  VectorParamsAs1DForOutWhenUnconnected=off
  wires:
  Saturation/1 -> current/1, Kt (Torque constant) Kt=Ke for an ideal square wave motor/1
  w angular speed/1 -> Ke (Torque constant)1/1
  ESC voltage/1 -> Sum/1
  Ke (Torque constant)1/1 -> Sum/2
  Kt (Torque constant) Kt=Ke for an ideal square wave motor/1 -> Electrical Torque/1
  Sum/1 -> 1/R/1
  1/R/1 -> Saturation/1  "current i"

== system digitaltwin1c/Motors/DC Motor 8/Mechanical part ==
  Static Friction Torque : Inport
  Electrical Torque : Inport  Port=2
  1/J Inertia constant : Gain  Gain=1/Motortwin8.J
  "Df viscous damping coefficient Dynamic Friction coefficient " : Gain  Gain=Motortwin8.Df
  Discrete-Time Integrator : DiscreteIntegrator  gainval=1  InitialCondition=IC.w8  SampleTime=octomodel.sampletime  ICPrevOutput=DiscIntNeverNeededParam  ICPrevScaledInput=DiscIntNeverNeededParam
  Gain : Gain  Gain=Motortwin8.cq
  Square : Math  Operator=square  SaturateOnIntegerOverflow=on
  Sum1 : Sum  Inputs=--+-
  w angular speed : Outport  VectorParamsAs1DForOutWhenUnconnected=off
  Torque : Outport  Port=2  VectorParamsAs1DForOutWhenUnconnected=off
  wires:
  Square/1 -> Gain/1
  Gain/1 -> Sum1/1, Torque/1
  Electrical Torque/1 -> Sum1/3
  Sum1/1 -> 1/J Inertia constant/1
  Discrete-Time Integrator/1 -> "Df viscous damping coefficient Dynamic Friction coefficient "/1, Square/1, w angular speed/1  "w angular speed"
  "Df viscous damping coefficient Dynamic Friction coefficient "/1 -> Sum1/4
  Static Friction Torque/1 -> Sum1/2
  1/J Inertia constant/1 -> Discrete-Time Integrator/1

== matlab function digitaltwin1c/lowsoc ==
  data: soc input; lowsoc output; threshold input
function lowsoc = fcn(soc,threshold)


if soc<threshold % less than one meter from the goal
    lowsoc=1;
else
    lowsoc=0;
end

== matlab function digitaltwin1c/arrival condition ==
  data: currentpos input; arrived output; dest input
function arrived = fcn(currentpos,dest)

result=norm(currentpos-dest);
if result<1 % less than one meter from the goal
    arrived=1;
else
    arrived=0;
end

== matlab function digitaltwin1c/Battery/MATLAB Function1 ==
  settings: updateMethod=DISCRETE  sampleTime=.2
  data: mu input; y output; sigma input
function y = addNoise(mu, sigma)

y = normrnd(mu, sigma);

== matlab function digitaltwin1c/Battery/MATLAB Function ==
  settings: updateMethod=DISCRETE  sampleTime=.2
  data: mu input; y output; sigma input
function y = addNoise(mu, sigma)

y = normrnd(mu, sigma);

== matlab function digitaltwin1c/Battery/MATLAB Function2 ==
  settings: updateMethod=DISCRETE  sampleTime=.2
  data: mu input; y output; sigma input
function y = addNoise(mu, sigma)

y = normrnd(mu, sigma);
